simulink model "FC1D"  (R2013a)
settings: Solver=ode3  StartTime=0.0  StopTime=tempo_sim  FixedStep=1e-4  MaxStep=1e-4
undefined symbols (not defined in the file): Aa, Ab, acc, beta, Cex, denC, denF, dx0n, dx0p, dxlimn, dxlimp, Fsn, Fsp, fv, Kd_pipe, Ke, Ki_pipe, Kp_pipe, Kva, Kvb, KvlkA, KvlkB, L, Mp, n, N_pipe, numC, numF, P0, pAo, pBo, pert_sen_amp, pert_sen_bias, pert_sen_freq, pert_step_degrau, pert_step_tempo, pert_trem_amp, pert_trem_ciclo, pert_trem_periodo, Polyn, Polyp, ps, pt, ref_sen_amp, ref_sen_bias, ref_sen_freq, ref_step_degrau, ref_step_tempo, ref_trem_amp, ref_trem_ciclo, ref_trem_periodo, sample_time, sel_atrito_hid, seletor_pert, sigbuilder_block, temp_pert, tipo_controlador, tipo_pert, tipo_ref, Un ... (+5)
libraries: sdolib x1, simulink x1
settings Model: Creator=RODRIGO  LastModifiedBy=Toshiba
settings SolverCC: ZeroCrossAlgorithm=Adaptive
settings OptimizationCC: ExpressionDepthLimit=2147483647
settings DebuggingCC: FcnCallInpInsideContextMsg=UseLocalSettings
settings GRTTargetCC: CombineOutputUpdateFcns=off  GRTInterface=on

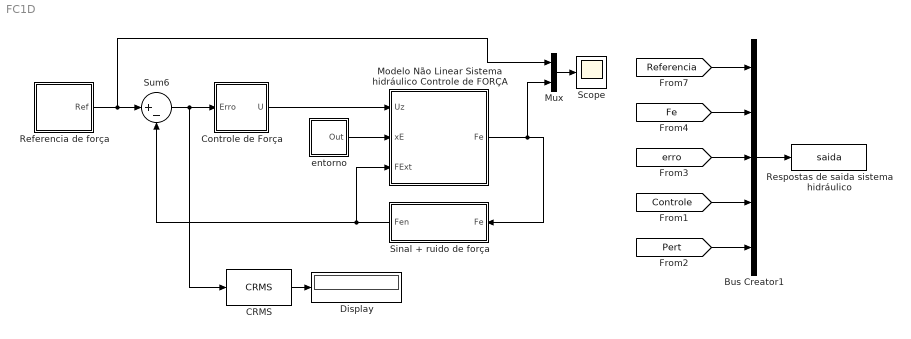
== system FC1D ==
  Bus Creator1 : BusCreator  Inputs=5
  CRMS : sdolib/RMS Blocks/CRMS
  Controle de Força : Subsystem
  Display : Display
  Modelo Não Linear Sistema hidráulico Controle de FORÇA : Subsystem
  Mux : Mux  Inputs=2
  Referencia de força : Subsystem
  Respostas de saida sistema hidráulico : ToWorkspace  VariableName=saida  SampleTime=sample_time  SaveFormat=Structure With Time
      settings: Decimation=decimation
  Scope : Scope
  Sinal + ruido de força : MATLAB Function  TreatAsAtomicUnit=on
  Sum6 : Sum  Inputs=|+-  SaturateOnIntegerOverflow=on  InputSameDT=on  OutDataTypeStr=Inherit: Same as first input
  entorno : Subsystem
  wires:
  [Referencia] -> Bus Creator1/1
  [Fe] -> Bus Creator1/2
  [erro] -> Bus Creator1/3
  [Controle] -> Bus Creator1/4
  entorno/1(Out) -> Modelo Não Linear Sistema hidráulico Controle de FORÇA/2(xE)
  Modelo Não Linear Sistema hidráulico Controle de FORÇA/1(Fe) -> Mux/2, Sinal + ruido de força/1(Fe)
  Sum6/1 -> CRMS/1, Controle de Força/1(Erro)
  Sinal + ruido de força/1(Fen) -> Sum6/2, Modelo Não Linear Sistema hidráulico Controle de FORÇA/3(FExt)
  Referencia de força/1(Ref) -> Mux/1, Sum6/1
  Controle de Força/1(U) -> Modelo Não Linear Sistema hidráulico Controle de FORÇA/1(Uz)
  Bus Creator1/1 -> Respostas de saida sistema hidráulico/1
  [Pert] -> Bus Creator1/5
  CRMS/1 -> Display/1
  Mux/1 -> Scope/1

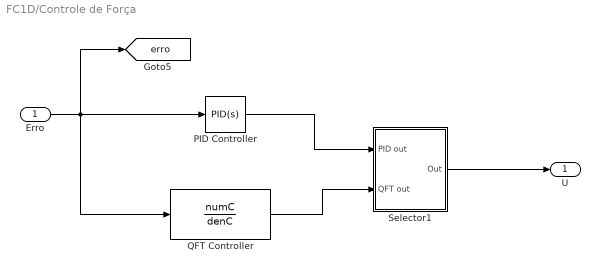
== system FC1D/Controle de Força ==
  Erro : Inport
  PID Controller : simulink/Continuous/PID Controller  Controller=PID  TimeDomain=Continuous-time  SampleTime=1  IntegratorMethod=Forward Euler  FilterMethod=Forward Euler  Form=Parallel  P=Kp_pipe  I=Ki_pipe  D=Kd_pipe  N=N_pipe  InitialConditionSource=internal  InitialConditionForIntegrator=0  InitialConditionForFilter=0  ExternalReset=none  LimitOutput=off  UpperSaturationLimit=inf  LowerSaturationLimit=-inf  LinearizeAsGain=on  AntiWindupMode=none  Kb=1  TrackingMode=off  Kt=1  PParamMin=[]  PParamMax=[]  IParamMin=[]  IParamMax=[]  DParamMin=[]  DParamMax=[]  NParamMin=[]  NParamMax=[]  KbParamMin=[]  KbParamMax=[]  KtParamMin=[]  KtParamMax=[]  POutMin=[]  POutMax=[]  IOutMin=[]  IOutMax=[]  DOutMin=[]  DOutMax=[]  NOutMin=[]  NOutMax=[]  KbOutMin=[]  KbOutMax=[]  KtOutMin=[]  KtOutMax=[]  IntegratorOutMin=[]  IntegratorOutMax=[]  FilterOutMin=[]  FilterOutMax=[]  SumOutMin=[]  SumOutMax=[]  SumI1OutMin=[]  SumI1OutMax=[]  SumI2OutMin=[]  SumI2OutMax=[]  SumI3OutMin=[]  SumI3OutMax=[]  SumDOutMin=[]  SumDOutMax=[]  SaturationOutMin=[]  SaturationOutMax=[]  IntegratorContinuousStateAttributes=''  IntegratorStateMustResolveToSignalObject=off  IntegratorRTWStateStorageClass=Auto  FilterContinuousStateAttributes=''  FilterStateMustResolveToSignalObject=off  FilterRTWStateStorageClass=Auto
  QFT Controller : TransferFcn  Numerator=numC  Denominator=denC
  Selector1 : Subsystem
  U : Outport
  tag scope: erro=global
  wires:
  Erro/1 -> [erro], PID Controller/1, QFT Controller/1
  PID Controller/1 -> Selector1/1(PID out)
  QFT Controller/1 -> Selector1/2(QFT out)
  Selector1/1(Out) -> U/1

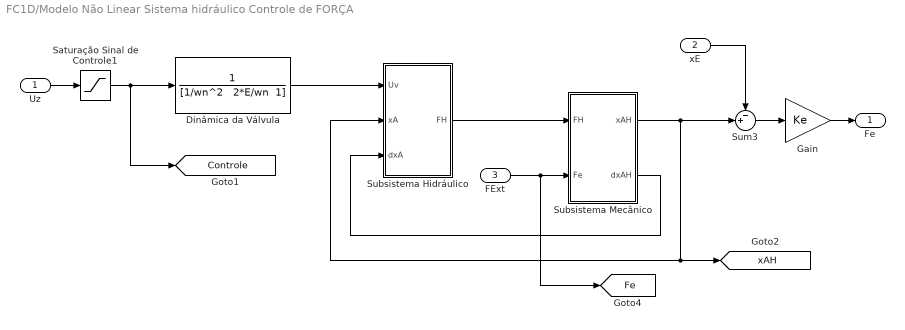
== system FC1D/Modelo Não Linear Sistema hidráulico Controle de FORÇA ==
  Uz : Inport
  xE : Inport  Port=2
  FExt : Inport  Port=3
  Dinâmica da Válvula : TransferFcn  Numerator=1  Denominator="[1/wn^2   2*E/wn  1]"
  Gain : Gain  Gain=Ke
  Saturação Sinal de Controle1 : Saturate  UpperLimit=10  LowerLimit=-10  LinearizeAsGain=off
  Subsistema Hidráulico : Subsystem
  Subsistema Mecânico : Subsystem
  Sum3 : Sum  Inputs=-+|
  Fe : Outport
  tag scope: Controle=global, Fe=global, xAH=global
  wires:
  Dinâmica da Válvula/1 -> Subsistema Hidráulico/1(Uv)
  Uz/1 -> Saturação Sinal de Controle1/1
  Subsistema Hidráulico/1(FH) -> Subsistema Mecânico/1(FH)
  Subsistema Mecânico/1(xAH) -> Sum3/2, Subsistema Hidráulico/2(xA), [xAH]
  Subsistema Mecânico/2(dxAH) -> Subsistema Hidráulico/3(dxA)
  Sum3/1 -> Gain/1
  Gain/1 -> Fe/1
  FExt/1 -> Subsistema Mecânico/2(Fe), [Fe]
  Saturação Sinal de Controle1/1 -> Dinâmica da Válvula/1, [Controle]
  xE/1 -> Sum3/1

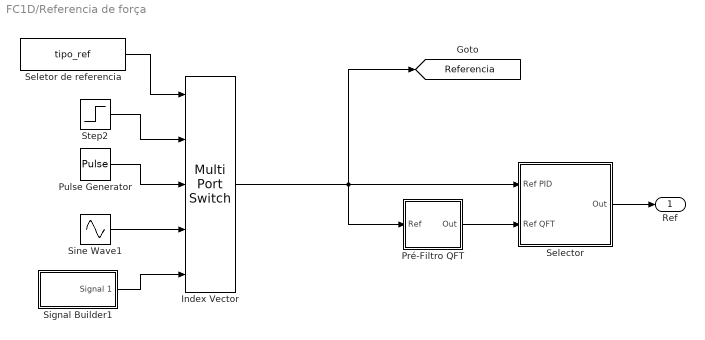
== system FC1D/Referencia de força ==
  Index Vector : MultiPortSwitch  Inputs=4
  Pré-Filtro QFT : Subsystem
  Pulse Generator : DiscretePulseGenerator  PulseType=Time based  Amplitude=ref_trem_amp  Period=ref_trem_periodo  PulseWidth=ref_trem_ciclo
  Selector : Subsystem
  Seletor de referencia : Constant  Value=tipo_ref
  Signal Builder1 : Subsystem  Tag=STV Subsys  LoadFcn=sigbuilder_block('load');  StartFcn=sigbuilder_block('start');  StopFcn=sigbuilder_block('stop');  ClipboardFcn=sigbuilder_block('clipboard');  mask(Sigbuilder block){}
      mask help: Create and generate interchangeable groups of signals whose waveforms are piecewise linear.
      mask init:
      | if ~strcmp(get_param(bdroot(gcbh),'SimulationStatus'),'stopped') tuvar = sigbuilder_block('maskInit'); end
      settings: CopyFcn=sigbuilder_block('copy');  DeleteFcn=sigbuilder_block('delete');  ModelCloseFcn=sigbuilder_block('modelClose');  PreSaveFcn=sigbuilder_block('preSave');  PauseFcn=sigbuilder_block('pause')  ContinueFcn=sigbuilder_block('continue')  NameChangeFcn=sigbuilder_block('namechange');  OpenFcn=sigbuilder_block('open',[228 103.5 550.5 399.75 ]);  CloseFcn=sigbuilder_block('close');
      mask Display: plot(0,0,100,100,[10,10,40,40,10],[80,20,20,80,80],[40,10],[50,50], [40,27,10],[65,72,56],[40,25,25,10],[28,28,43,43]);
  Sine Wave1 : Sin  Amplitude=ref_sen_amp  Bias=ref_sen_bias  Frequency=ref_sen_freq  SampleTime=0
  Step2 : Step  Time=ref_step_tempo  After=ref_step_degrau  SampleTime=0
  Ref : Outport
  tag scope: Referencia=global
  wires:
  Signal Builder1/1(Signal 1) -> Index Vector/5
  Sine Wave1/1 -> Index Vector/4
  Pulse Generator/1 -> Index Vector/3
  Step2/1 -> Index Vector/2
  Seletor de referencia/1 -> Index Vector/1
  Index Vector/1 -> Selector/1(Ref PID), Pré-Filtro QFT/1(Ref), [Referencia]
  Pré-Filtro QFT/1(Out) -> Selector/2(Ref QFT)
  Selector/1(Out) -> Ref/1

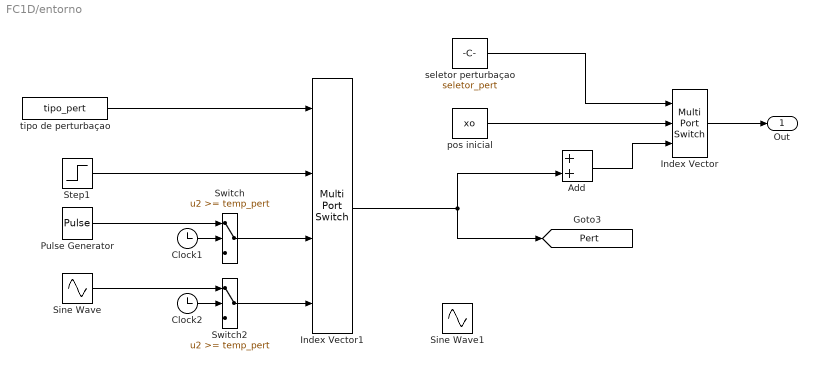
== system FC1D/entorno ==
  Add : Sum
  Clock1 : Clock
  Clock2 : Clock
  Index Vector : MultiPortSwitch  DataPortOrder=Zero-based contiguous  Inputs=2
  Index Vector1 : MultiPortSwitch
  Pulse Generator : DiscretePulseGenerator  PulseType=Time based  Amplitude=pert_trem_amp  Period=pert_trem_periodo  PulseWidth=pert_trem_ciclo
  Sine Wave : Sin  Amplitude=pert_sen_amp  Bias=pert_sen_bias  Frequency=pert_sen_freq  SampleTime=0
  Sine Wave1 : Sin  Amplitude=pert_sen_amp  Bias=pert_sen_bias  Frequency=pert_sen_freq  SampleTime=0
  Step1 : Step  Time=pert_step_tempo  After=pert_step_degrau  SampleTime=0
  Switch : Switch  Threshold=temp_pert
  Switch2 : Switch  Threshold=temp_pert
  pos inicial : Constant  Value=xo
  seletor perturbaçao : Constant  Value=seletor_pert
  tipo de perturbaçao : Constant  Value=tipo_pert
  Out : Outport
  tag scope: Pert=global
  wires:
  Index Vector/1 -> Out/1
  seletor perturbaçao/1 -> Index Vector/1
  Step1/1 -> Index Vector1/2
  tipo de perturbaçao/1 -> Index Vector1/1
  Clock1/1 -> Switch/2
  Pulse Generator/1 -> Switch/1
  Switch/1 -> Index Vector1/3
  Clock2/1 -> Switch2/2
  Switch2/1 -> Index Vector1/4
  Sine Wave/1 -> Switch2/1
  pos inicial/1 -> Index Vector/2
  Index Vector1/1 -> [Pert], Add/2
  Add/1 -> Index Vector/3

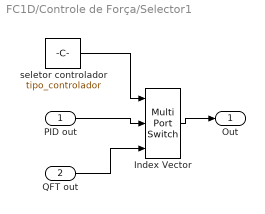
== system FC1D/Controle de Força/Selector1 ==
  PID out : Inport
  QFT out : Inport  Port=2
  Index Vector : MultiPortSwitch  Inputs=2
  seletor controlador : Constant  Value=tipo_controlador
  Out : Outport
  wires:
  Index Vector/1 -> Out/1
  seletor controlador/1 -> Index Vector/1
  PID out/1 -> Index Vector/2
  QFT out/1 -> Index Vector/3

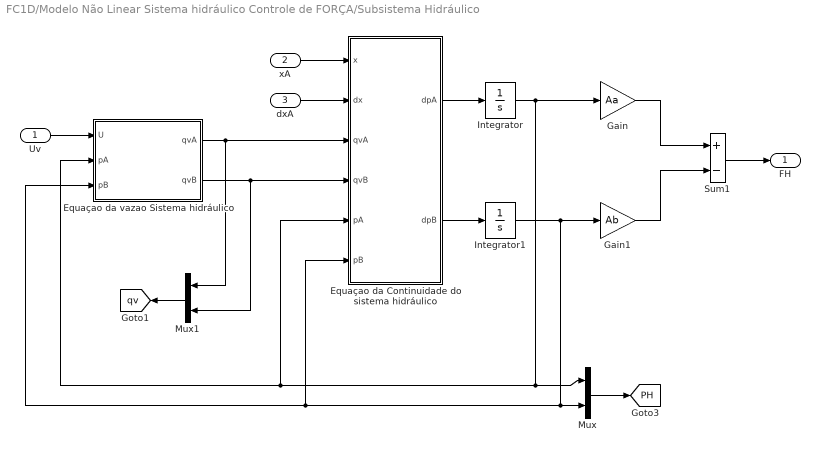
== system FC1D/Modelo Não Linear Sistema hidráulico Controle de FORÇA/Subsistema Hidráulico ==
  Uv : Inport
  xA : Inport  Port=2
  dxA : Inport  Port=3
  Equaçao da Continuidade do sistema hidráulico : MATLAB Function  TreatAsAtomicUnit=on
  Equaçao da vazao Sistema hidráulico : MATLAB Function  TreatAsAtomicUnit=on
  Gain : Gain  Gain=Aa  SaturateOnIntegerOverflow=on  OutDataTypeStr=Inherit: Same as input  ParamDataTypeStr=Inherit: Same as input
  Gain1 : Gain  Gain=Ab  SaturateOnIntegerOverflow=on  OutDataTypeStr=Inherit: Same as input  ParamDataTypeStr=Inherit: Same as input
  Integrator : Integrator  InitialCondition=pAo
  Integrator1 : Integrator  InitialCondition=pBo
  Mux : Mux  Inputs=2
  Mux1 : Mux  Inputs=2
  Sum1 : Sum  Inputs=+-  SaturateOnIntegerOverflow=on  InputSameDT=on  OutDataTypeStr=Inherit: Same as first input
  FH : Outport
  tag scope: PH=global, qv=global
  wires:
  Sum1/1 -> FH/1
  Gain1/1 -> Sum1/2
  Gain/1 -> Sum1/1
  Integrator/1 -> Gain/1, Equaçao da vazao Sistema hidráulico/2(pA), Equaçao da Continuidade do sistema hidráulico/5(pA), Mux/1
  Integrator1/1 -> Gain1/1, Equaçao da vazao Sistema hidráulico/3(pB), Equaçao da Continuidade do sistema hidráulico/6(pB), Mux/2
  Equaçao da Continuidade do sistema hidráulico/2(dpB) -> Integrator1/1
  Equaçao da Continuidade do sistema hidráulico/1(dpA) -> Integrator/1
  xA/1 -> Equaçao da Continuidade do sistema hidráulico/1(x)
  dxA/1 -> Equaçao da Continuidade do sistema hidráulico/2(dx)
  Uv/1 -> Equaçao da vazao Sistema hidráulico/1(U)
  Equaçao da vazao Sistema hidráulico/2(qvB) -> Mux1/2, Equaçao da Continuidade do sistema hidráulico/4(qvB)
  Equaçao da vazao Sistema hidráulico/1(qvA) -> Mux1/1, Equaçao da Continuidade do sistema hidráulico/3(qvA)
  Mux/1 -> [PH]
  Mux1/1 -> [qv]

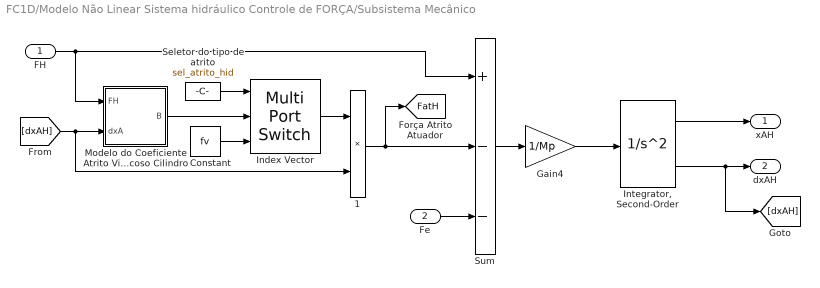
== system FC1D/Modelo Não Linear Sistema hidráulico Controle de FORÇA/Subsistema Mecânico ==
  FH : Inport
  Fe : Inport  Port=2
  "    1" : Product  SaturateOnIntegerOverflow=on  OutDataTypeStr=Inherit: Same as first input
  Constant : Constant  Value=fv
  Gain4 : Gain  Gain=1/Mp  SaturateOnIntegerOverflow=on  OutDataTypeStr=Inherit: Same as input  ParamDataTypeStr=Inherit: Same as input
  Index Vector : MultiPortSwitch  Inputs=2
  "Integrator, Second-Order" : SecondOrderIntegrator  ICX=xo  LimitX=on  UpperLimitX=L  LowerLimitX=0
  "Modelo do Coeficiente Atrito Viscoso Cilindro " : Subsystem
  Seletor do tipo de atrito : Constant  Value=sel_atrito_hid
  Sum : Sum  Inputs=+--  SaturateOnIntegerOverflow=on  InputSameDT=on  OutDataTypeStr=Inherit: Same as first input
  xAH : Outport
  dxAH : Outport  Port=2
  tag scope: FatH=global
  wires:
  "Integrator, Second-Order"/1 -> xAH/1
  Sum/1 -> Gain4/1
  Fe/1 -> Sum/3
  FH/1 -> Sum/1, "Modelo do Coeficiente Atrito Viscoso Cilindro "/1(FH)
  [dxAH] -> "Modelo do Coeficiente Atrito Viscoso Cilindro "/2(dxA), "    1"/2
  "Modelo do Coeficiente Atrito Viscoso Cilindro "/1(B) -> Index Vector/2
  "    1"/1 -> [FatH], Sum/2
  "Integrator, Second-Order"/2 -> dxAH/1, [dxAH]
  Gain4/1 -> "Integrator, Second-Order"/1
  Index Vector/1 -> "    1"/1
  Constant/1 -> Index Vector/3
  Seletor do tipo de atrito/1 -> Index Vector/1

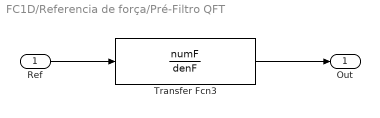
== system FC1D/Referencia de força/Pré-Filtro QFT ==
  Ref : Inport
  Transfer Fcn3 : TransferFcn  Numerator=numF  Denominator=denF
  Out : Outport
  wires:
  Ref/1 -> Transfer Fcn3/1
  Transfer Fcn3/1 -> Out/1

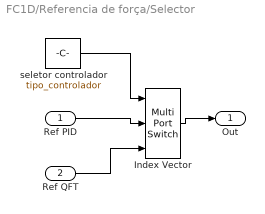
== system FC1D/Referencia de força/Selector ==
  Ref PID : Inport
  Ref QFT : Inport  Port=2
  Index Vector : MultiPortSwitch  Inputs=2
  seletor controlador : Constant  Value=tipo_controlador
  Out : Outport
  wires:
  Ref QFT/1 -> Index Vector/3
  Ref PID/1 -> Index Vector/2
  seletor controlador/1 -> Index Vector/1
  Index Vector/1 -> Out/1

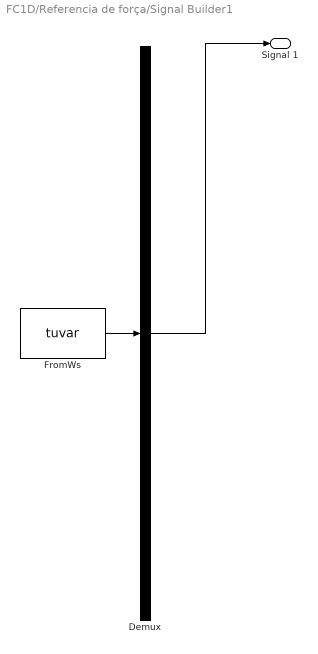
== system FC1D/Referencia de força/Signal Builder1 ==
  Demux : Demux  Tag=STV Demux  Outputs=1
  FromWs : FromWorkspace  Tag=STV FromWs  VariableName=tuvar  SampleTime=0
      SigBuilderData=|
      | common.afterFinalStr = 'Extrapolate'
      | common.sampleTime = 0
      | dataSet.timeRange = [0 30]
      | dataSet.name = 'Group 1'
      | sbobj.Groups.Name = 'Group 1'
      | sbobj.Groups.Signals.Name = 'Signal 1'
      | sbobj.Groups.Signals.XData = [0 1 1 4 4 7 7 10 10 13 13 14 16 16 17 20 30]
      | sbobj.Groups.Signals.YData = [-0.002 -0.002 1000 1000 -3000 -3000 3000 3000 9000 9000 7000 7000 2000 -5800 -5800 1000 1000]
      | sbobj.Groups.TimeRange = [0 30]
  Signal 1 : Outport  Tag=STV Outport
  wires:
  FromWs/1 -> Demux/1
  Demux/1 -> Signal 1/1

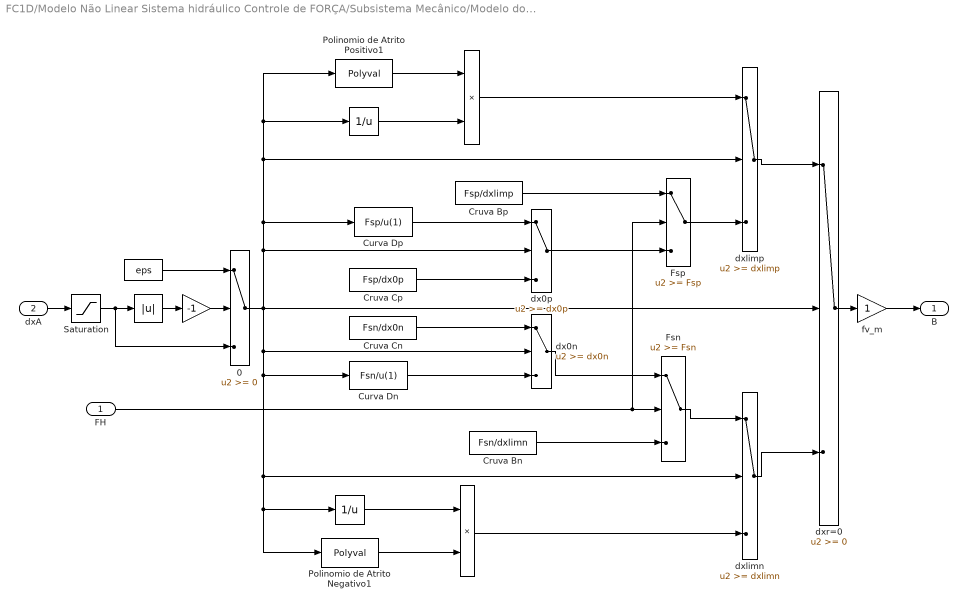
== system FC1D/Modelo Não Linear Sistema hidráulico Controle de FORÇA/Subsistema Mecânico/Modelo do Coeficiente Atrito Viscoso Cilindro  ==
  FH : Inport
  dxA : Inport  Port=2
  " " : Abs  SaturateOnIntegerOverflow=on
  "  " : Gain  Gain=-1  SaturateOnIntegerOverflow=on  OutDataTypeStr=Inherit: Same as input  ParamDataTypeStr=Inherit: Same as input
  "   " : Product  SaturateOnIntegerOverflow=on  OutDataTypeStr=Inherit: Same as first input
  "     " : Math  Operator=reciprocal  SaturateOnIntegerOverflow=on
  "      " : Product  SaturateOnIntegerOverflow=on  OutDataTypeStr=Inherit: Same as first input
  "        " : Math  Operator=reciprocal  SaturateOnIntegerOverflow=on
  "                 " : Constant  Value=eps
  0 : Switch  SaturateOnIntegerOverflow=on
  Cruva Bn : Constant  Value=Fsn/dxlimn
  Cruva Bp : Constant  Value=Fsp/dxlimp
  Cruva Cn : Constant  Value=Fsn/dx0n
  Cruva Cp : Constant  Value=Fsp/dx0p
  Curva Dn : Fcn  Expr=Fsn/u(1)
  Curva Dp : Fcn  Expr=Fsp/u(1)
  Fsn : Switch  Threshold=Fsn  SaturateOnIntegerOverflow=on
  Fsp : Switch  Threshold=Fsp  SaturateOnIntegerOverflow=on
  Polinomio de Atrito Negativo1 : Polyval  Coefs=Polyn
  Polinomio de Atrito Positivo1 : Polyval  Coefs=Polyp
  Saturation : Saturate  UpperLimit=0.8  LowerLimit=-0.8
  dx0n : Switch  Threshold=dx0n  SaturateOnIntegerOverflow=on
  dx0p : Switch  Threshold=dx0p  SaturateOnIntegerOverflow=on
  dxlimn : Switch  Threshold=dxlimn  SaturateOnIntegerOverflow=on
  dxlimp : Switch  Threshold=dxlimp  SaturateOnIntegerOverflow=on
  dxr=0 : Switch  SaturateOnIntegerOverflow=on
  fv_m : Gain  SaturateOnIntegerOverflow=on  OutDataTypeStr=Inherit: Same as input  ParamDataTypeStr=Inherit: Same as input
  B : Outport
  wires:
  Polinomio de Atrito Positivo1/1 -> "   "/1
  Polinomio de Atrito Negativo1/1 -> "      "/2
  Saturation/1 -> 0/3, " "/1
  dxA/1 -> Saturation/1
  fv_m/1 -> B/1
  "  "/1 -> 0/2
  "     "/1 -> "   "/2
  0/1 -> dxr=0/2, dx0n/2, Polinomio de Atrito Negativo1/1, "        "/1, dxlimn/2, Curva Dn/1, Polinomio de Atrito Positivo1/1, "     "/1, dxlimp/2, Curva Dp/1, dx0p/2
  dxlimp/1 -> dxr=0/1
  "        "/1 -> "      "/1
  Fsp/1 -> dxlimp/3
  Fsn/1 -> dxlimn/1
  dxr=0/1 -> fv_m/1
  "   "/1 -> dxlimp/1
  "      "/1 -> dxlimn/3
  dxlimn/1 -> dxr=0/3
  dx0p/1 -> Fsp/3
  Curva Dp/1 -> dx0p/1
  Cruva Cp/1 -> dx0p/3
  dx0n/1 -> Fsn/1
  Cruva Bn/1 -> Fsn/3
  Curva Dn/1 -> dx0n/3
  Cruva Cn/1 -> dx0n/1
  FH/1 -> Fsn/2, Fsp/2
  Cruva Bp/1 -> Fsp/1
  " "/1 -> "  "/1
  "                 "/1 -> 0/1

== matlab function FC1D/Sinal + ruido de força ==
  data: Fe input; Fen output
function Fen = fcn(Fe)

Fen = Fe + 0.1*randn(1,1);

== matlab function FC1D/Modelo Não Linear Sistema hidráulico Controle de FORÇA/Subsistema Hidráulico/Equaçao da vazao Sistema hidráulico ==
  data U settings: updateMethod=SF_CONTINUOUS_TIME_DATA
  data qvA settings: updateMethod=SF_CONTINUOUS_TIME_DATA
  data qvB settings: updateMethod=SF_CONTINUOUS_TIME_DATA
  data: U input; qvA output; qvB output; Un parameter; Kva parameter; Kvb parameter; KvlkA parameter; KvlkB parameter; ps parameter; pt parameter; pA input; pB input
function [qvA , qvB] = fcn(U, Un, Kva, Kvb, KvlkA, KvlkB, ps, pt, pA, pB)

if U>=0,
    qvA = (Kva*(U/Un) + KvlkA) * sign(ps-pA)*sqrt(abs(ps-pA)) - KvlkA*sign(pA-pt)*sqrt(abs(pA-pt)) ;
    qvB = (Kvb*(U/Un) + KvlkB) * sign(pB-pt)*sqrt(abs(pB-pt)) - KvlkB*sign(ps-pB)*sqrt(abs(ps-pB)) ;
else qvA = KvlkA*sign(ps-pA)*sqrt(abs(ps-pA)) - (Kva*(abs(U)/Un) + KvlkA) * sign(pA-pt)*sqrt(abs(pA-pt));
     qvB = KvlkB*sign(pB-pt)*sqrt(abs(pB-pt)) - (Kvb*(abs(U)/Un) + KvlkB) * sign(ps-pB)*sqrt(abs(ps-pB));
end

== matlab function FC1D/Modelo Não Linear Sistema hidráulico Controle de FORÇA/Subsistema Hidráulico/Equaçao da Continuidade do sistema hidráulico ==
  data: x input; dpA output; dpB output; dx input; qvA input; qvB input; pA input; pB input; Cex parameter; V0A parameter; V0B parameter; Aa parameter; Ab parameter; L parameter; beta parameter; n parameter; V0 parameter; P0 parameter; acc parameter
function [dpA,dpB] = fcn(x, dx, qvA, qvB, pA, pB, Cex, V0A, V0B, Aa, Ab, L, beta, n, V0, P0, acc)

pC = pA - pB;   % Pressao de carga [Pa]

qvex = Cex * pC;
dpa = 0;
dpb = 0;

if acc == 0,
%       /              \
%       |     beta     | /                    \
% dpA = | ------------ | | qvA - Aa*dx - qvex | 
%       |  Va0 + Aa*x  | \                    /
%       \              /
      
dpa = (beta/(V0A + Aa*x)) * (qvA - Aa*dx - qvex);

%       /                  \
%       |     beta         | /                    \
% dpB = | ---------------- | | Ab*dx + qvex - qvB | 
%       | Vb0 + Ab*(L - x) | \                    /
%       \                  /
      
dpb = (beta/(V0B + Ab*(L-x))) * (Ab*dx + qvex - qvB);

elseif acc == 1,
    
CA_A  = (V0A + Aa*x) / beta;                      % Capacitancia hidráulica do atuador [m^3/Pa]
CAC_A = (V0*P0^(1/n))/(n* (pA+1e5)^((n+1)/n));     % Capacitancia hidráulica do acumulador [m^3/Pa]
CA_B  = (V0B + Ab*(L-x)) / beta;                  % Capacitancia hidráulica do atuador [m^3/Pa]
CAC_B = (V0*P0^(1/n))/(n* (pB+1e5)^((n+1)/n));     % Capacitancia hidráulica do acumulador [m^3/Pa]

CT_A  = CA_A + CAC_A;                              % Capacitancia total em A
CT_B  = CA_B + CAC_B;                              % Capacitancia total em B 


%       /        \
%       |   1    | /                    \
% dpA = | ------ | | qvA - Aa*dx - qvex | 
%       |  CT_A  | \                    /
%       \        /
      
dpa = CT_A^-1 * (qvA - Aa*dx - qvex);

%       /        \
%       |   1    | /                    \
% dpB = | ------ | | Ab*dx + qvex - qvB | 
%       |  CT_B  | \                    /
%       \        /
      
dpb = CT_B^-1 * (Ab*dx + qvex - qvB);
end

dpA = dpa;
dpB = dpb;
